simulink model "lab5model"  (R2022b)
settings: Solver=VariableStepAuto  StartTime=0.0  StopTime=50  RelTol=1e-3
undefined symbols (not defined in the file): A, b, c, M
settings Model: Creator=Andrzej  LastModifiedBy=Andrzej
settings DataIOCC: SaveFormat=StructureWithTime  ReturnWorkspaceOutputs=off

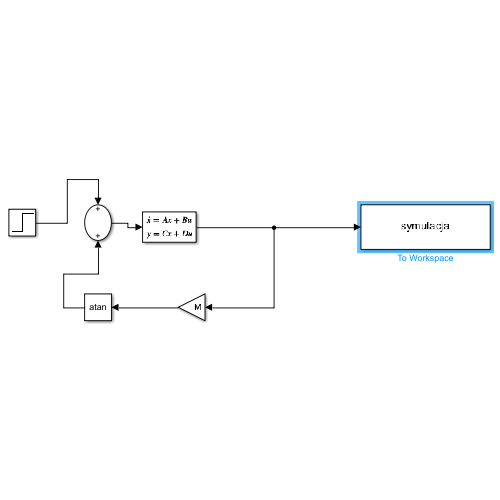
[thumbnail: Simulink's stored preview of the top-level diagram]
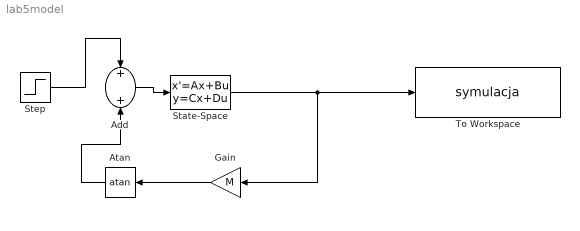
== system lab5model ==
  Add : Sum
  Atan : Trigonometry  Operator=atan
  Gain : Gain  Gain=M
  State-Space : StateSpace  A=A  B=b  C=c  D=[0]  InitialCondition=0
  Step : Step  Time=0  SampleTime=0
  To Workspace : ToWorkspace  VariableName=symulacja  SampleTime=-1
      settings: Save2DSignal=2-D array (concatenate along first dimension)
  wires:
  Step/1 -> Add/1
  Gain/1 -> Atan/1
  Atan/1 -> Add/2
  Add/1 -> State-Space/1
  State-Space/1 -> To Workspace/1, Gain/1
